simulink model "simulinkModel"  (R2015a)
settings: Solver=ode45  StartTime=0.0  StopTime=10.0  RelTol=1e-3
settings Model: Creator=anatole  LastModifiedBy=anatole

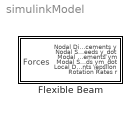
== system simulinkModel ==
  Flexible Beam : Subsystem

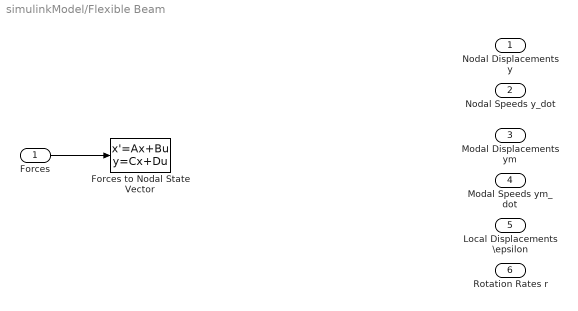
== system simulinkModel/Flexible Beam ==
  Forces : Inport
  Forces to Nodal State Vector : StateSpace  X0=0
  Nodal Displacements y : Outport
  Nodal Speeds y_dot : Outport  Port=2
  Modal Displacements ym : Outport  Port=3
  Modal Speeds ym_dot : Outport  Port=4
  Local Displacements \epsilon : Outport  Port=5
  Rotation Rates r : Outport  Port=6
  wires:
  Forces/1 -> Forces to Nodal State Vector/1
